simulink model "soar_interp_test"  (R2018b)
settings: Solver=FixedStepAuto  StartTime=0.0  StopTime=30  FixedStep=soarParams.sample_time_s  RelTol=1e-3
values from neighbouring files (symbols this model uses):
  hw_ic = xopt(8:10,1)    [soar_interp_test_init.m]
  quat_ic = xopt(1:4,1)    [soar_interp_test_init.m]
  w_ic = J\xopt(5:7,1)    [soar_interp_test_init.m]
undefined symbols (not defined in the file or in its folder): simParams, soarParams, sopt, uopt, xopt
libraries: simulink x2, quat_degerr_lib x1, soar_interp x1
settings Model: Creator=Taylor  LastModifiedBy=Taylor

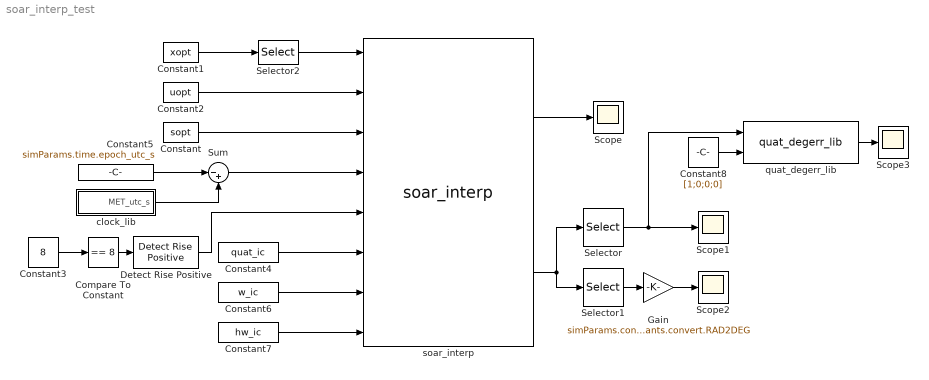
== system soar_interp_test ==
  Compare To Constant : simulink/Logic and Bit Operations/Compare To Constant  relop===  const=8  OutDataTypeStr=boolean
  Constant : Constant  Value=sopt
  Constant1 : Constant  Value=xopt
  Constant2 : Constant  Value=uopt
  Constant3 : Constant  Value=8  OutDataTypeStr=uint8
  Constant4 : Constant  Value=quat_ic
  Constant5 : Constant  Value=simParams.time.epoch_utc_s  SampleTime=-1
  Constant6 : Constant  Value=w_ic
  Constant7 : Constant  Value=hw_ic
  Constant8 : Constant  Value=[1;0;0;0]
  Detect Rise Positive : simulink/Logic and Bit Operations/Detect Rise Positive  vinit=0  OutDataTypeStr=boolean
  Gain : Gain  Gain=simParams.constants.convert.RAD2DEG
  Scope{,1..3} (4 alike) : Scope
  Selector : Selector  InputPortWidth=10  IndexOptions=Index vector (dialog)  Indices=[1 2 3 4]  OutputSizes=1
  Selector1 : Selector  InputPortWidth=10  IndexOptions=Index vector (dialog)  Indices=[5 6 7]  OutputSizes=1
  Selector2 : Selector  NumberOfDimensions=2  InputPortWidth=3  IndexOptions=Select all,Index vector (dialog)  Indices=[1 3],10  OutputSizes=1,1
  Sum : Sum  Inputs=|-+
  clock_lib : Subsystem
  quat_degerr_lib : quat_degerr_lib/quat_degerr_lib  SystemSampleTime=-1
  soar_interp : soar_interp/soar_interp  SystemSampleTime=-1
  wires:
  Constant/1 -> soar_interp/3
  Constant1/1 -> Selector2/1
  Constant2/1 -> soar_interp/2
  Detect Rise Positive/1 -> soar_interp/5
  Constant5/1 -> Sum/1
  clock_lib/1(MET_utc_s) -> Sum/2
  Sum/1 -> soar_interp/4
  Constant4/1 -> soar_interp/6
  Constant6/1 -> soar_interp/7
  Constant7/1 -> soar_interp/8
  soar_interp/1 -> Scope/1
  soar_interp/2 -> Selector/1, Selector1/1
  Selector/1 -> quat_degerr_lib/1, Scope1/1
  Selector1/1 -> Gain/1
  Selector2/1 -> soar_interp/1
  Compare To Constant/1 -> Detect Rise Positive/1
  Constant3/1 -> Compare To Constant/1
  Gain/1 -> Scope2/1
  Constant8/1 -> quat_degerr_lib/2
  quat_degerr_lib/1 -> Scope3/1

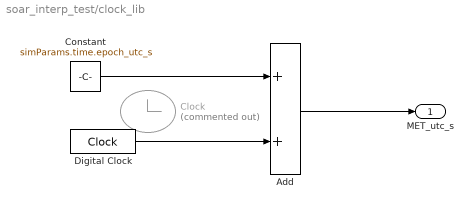
== system soar_interp_test/clock_lib ==
  Add : Sum
  Clock : Clock  Commented=on
  Constant : Constant  Value=simParams.time.epoch_utc_s
  Digital Clock : DigitalClock  SampleTime=soarParams.sample_time_s
  MET_utc_s : Outport
  wires:
  Digital Clock/1 -> Add/2
  Constant/1 -> Add/1
  Add/1 -> MET_utc_s/1
